simulink model "VehicleModelwithLateralController_comp"  (R2019b)
settings: Solver=FixedStepAuto  StartTime=0.0  StopTime=60  FixedStep=0.05  RelTol=1e-3
values from neighbouring files (symbols this model uses):
  Iz = car.iz    [Vehicle_Parameters_and_initial_state_comp.m]    (also in sfun_LQRwithFF_YC_2DOF.m; sfun_MPC_YC_2DOF.m; sfun_MPC_deltaU_YC_2DOF.m; sfun_MPC_deltaU_softcon_YC_2DOF.m)
  Kyf = car.kyf    [Vehicle_Parameters_and_initial_state_comp.m]    (also in sfun_LQRwithFF_YC_2DOF.m; sfun_MPC_YC_2DOF.m; sfun_MPC_deltaU_YC_2DOF.m; sfun_MPC_deltaU_softcon_YC_2DOF.m)
  Kyr = car.kyr    [Vehicle_Parameters_and_initial_state_comp.m]    (also in sfun_LQRwithFF_YC_2DOF.m; sfun_MPC_YC_2DOF.m; sfun_MPC_deltaU_YC_2DOF.m; sfun_MPC_deltaU_softcon_YC_2DOF.m)
  lf = car.lf    [Vehicle_Parameters_and_initial_state_comp.m]    (also in sfun_LQRwithFF_YC_2DOF.m; sfun_MPC_YC_2DOF.m; sfun_MPC_deltaU_YC_2DOF.m; sfun_MPC_deltaU_softcon_YC_2DOF.m)
  lr = car.lr    [Vehicle_Parameters_and_initial_state_comp.m]    (also in sfun_LQRwithFF_YC_2DOF.m; sfun_MPC_YC_2DOF.m; sfun_MPC_deltaU_YC_2DOF.m; sfun_MPC_deltaU_softcon_YC_2DOF.m)
  m = car.m    [Vehicle_Parameters_and_initial_state_comp.m]    (also in sfun_LQRwithFF_YC_2DOF.m; sfun_MPC_YC_2DOF.m; sfun_MPC_deltaU_YC_2DOF.m = 1; sfun_MPC_deltaU_softcon_YC_2DOF.m)
  Ta = a11+a22    [sfun_MPC_deltaU_softcon_YC_2DOF.m]
  Vx = 72/3.6    (= 20)    [Vehicle_Parameters_and_initial_state_comp.m]    (also in sfun_LQRwithFF_YC_2DOF.m = VehIniSt.xd; sfun_MPC_YC_2DOF.m = VehIniSt.xd; sfun_MPC_deltaU_YC_2DOF.m = VehIniSt.xd; sfun_MPC_deltaU_softcon_YC_2DOF.m = VehIniSt.xd)
  X_up = 140    [Vehicle_Parameters_and_initial_state_comp.m]
undefined symbols (not defined in the file or in its folder): car, Tra, VehIniSt
libraries: simulink x2
settings Model: Creator=pc  LastModifiedBy=YC

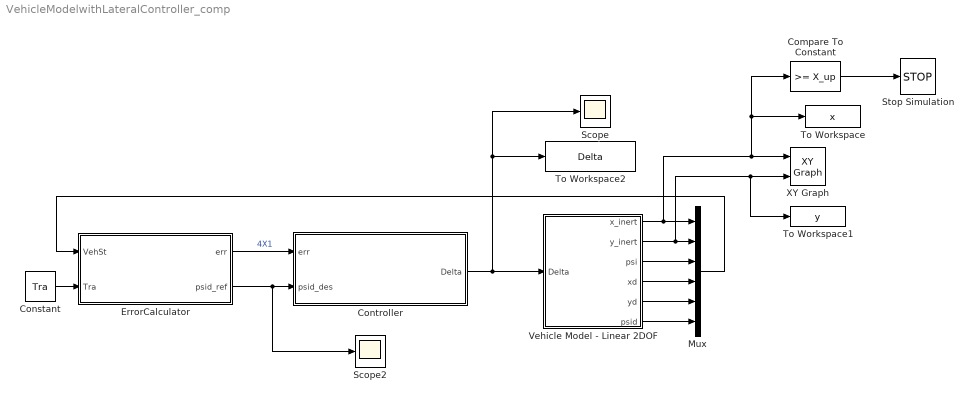
== system VehicleModelwithLateralController_comp ==
  Compare To Constant : simulink/Logic and Bit Operations/Compare To Constant  relop=>=  const=X_up  OutDataTypeStr=boolean
  Constant : Constant  Value=Tra
  Controller : Subsystem  Variant=on
  ErrorCalculator : Subsystem  Variant=on
  Mux : Mux  Inputs=6
  Scope : Scope
  Scope2 : Scope
  Stop Simulation : Stop
  To Workspace : ToWorkspace  VariableName=x  SampleTime=-1
  To Workspace1 : ToWorkspace  VariableName=y  SampleTime=-1
  To Workspace2 : ToWorkspace  VariableName=Delta  SampleTime=-1
  Vehicle Model - Linear 2DOF : Subsystem  mask{Ar=[-(2*Kyf+2*Kyr)/m/Vx,-Vx-(2*Kyf*lf-2*Kyr*lr)/m/Vx;-(2*Kyf*lf-2*Kyr*lr)/Iz/Vx,-(2*Kyf*lf.^2+2*Kyr*lr.^2)/Iz/Vx], Br=[2*Kyf/m;2*Kyf*lf/Iz], Cr=[1,0;0,1], Dr=[0;0]}
  XY Graph : simulink/Sinks/XY Graph  xmin=0  xmax=150  ymin=-1  ymax=4  st=-1
  wires:
  Compare To Constant/1 -> Stop Simulation/1
  Constant/1 -> ErrorCalculator/2(Tra)
  ErrorCalculator/1(err) -> Controller/1(err)  "4X1"
  ErrorCalculator/2(psid_ref) -> Scope2/1, Controller/2(psid_des)
  Controller/1(Delta) -> Vehicle Model - Linear 2DOF/1(Delta), Scope/1, To Workspace2/1
  Vehicle Model - Linear 2DOF/1(x_inert) -> Compare To Constant/1, To Workspace/1, XY Graph/1, Mux/1
  Vehicle Model - Linear 2DOF/2(y_inert) -> To Workspace1/1, XY Graph/2, Mux/2
  Vehicle Model - Linear 2DOF/3(psi) -> Mux/3
  Vehicle Model - Linear 2DOF/4(xd) -> Mux/4
  Vehicle Model - Linear 2DOF/5(yd) -> Mux/5
  Vehicle Model - Linear 2DOF/6(psid) -> Mux/6
  Mux/1 -> ErrorCalculator/1(VehSt)

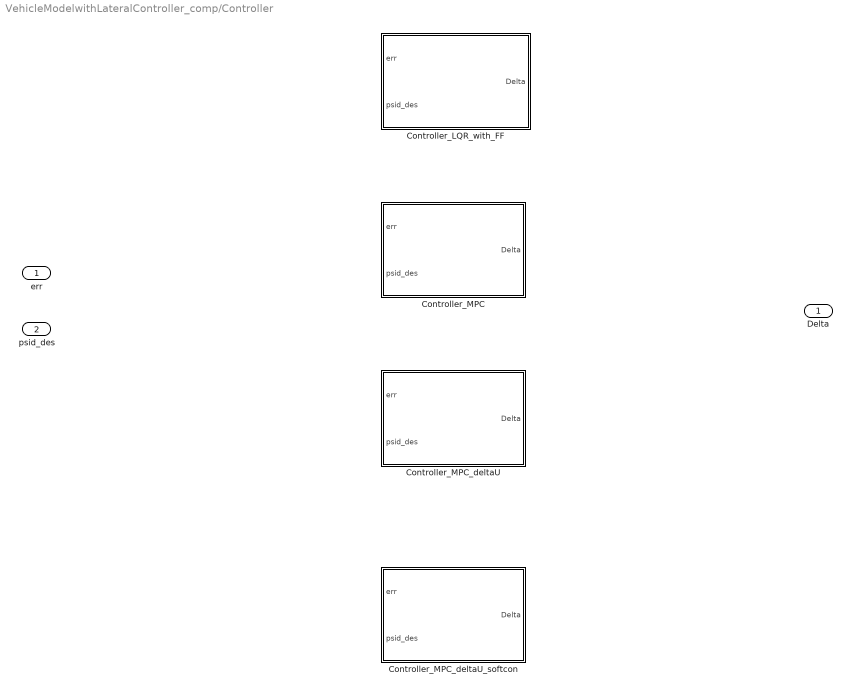
== system VehicleModelwithLateralController_comp/Controller ==
  err : Inport
  psid_des : Inport  Port=2
  Controller_LQR_with_FF : Subsystem  VariantControl=Controller_mode==1
  Controller_MPC : Subsystem  VariantControl=Controller_mode==2
  Controller_MPC_deltaU : Subsystem  VariantControl=Controller_mode==3
  Controller_MPC_deltaU_softcon : Subsystem  VariantControl=Controller_mode==4
  Delta : Outport

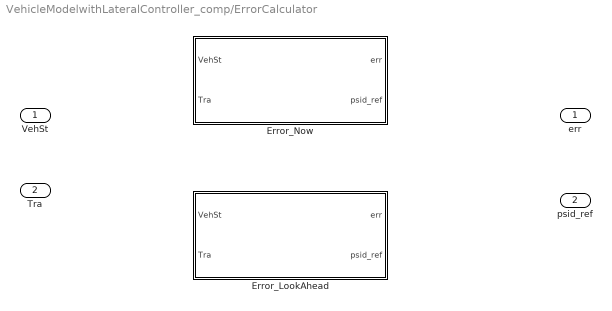
== system VehicleModelwithLateralController_comp/ErrorCalculator ==
  VehSt : Inport
  Tra : Inport  Port=2
  Error_LookAhead : Subsystem  VariantControl=Error_Mode==1
  Error_Now : Subsystem  VariantControl=Error_Mode==0
  err : Outport
  psid_ref : Outport  Port=2

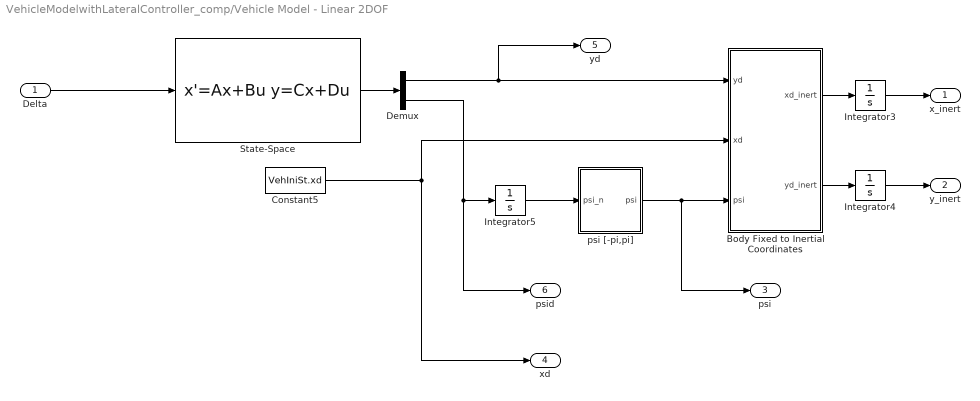
== system VehicleModelwithLateralController_comp/Vehicle Model - Linear 2DOF ==
  Delta : Inport
  Body Fixed to Inertial Coordinates : Subsystem
  Constant5 : Constant  Value=VehIniSt.xd
  Demux : Demux  Outputs=2
  Integrator3 : Integrator  InitialCondition=VehIniSt.x0
  Integrator4 : Integrator  InitialCondition=VehIniSt.y0
  Integrator5 : Integrator  InitialCondition=VehIniSt.psi0
  State-Space : StateSpace  A=Ar  B=Br  C=Cr  D=Dr  InitialCondition=0
  psi [-pi,pi] : MATLAB Function  TreatAsAtomicUnit=on
  x_inert : Outport
  y_inert : Outport  Port=2
  psi : Outport  Port=3
  xd : Outport  Port=4
  yd : Outport  Port=5
  psid : Outport  Port=6
  wires:
  Demux/2 -> Integrator5/1, psid/1
  State-Space/1 -> Demux/1
  Demux/1 -> yd/1, Body Fixed to Inertial Coordinates/1(yd)
  Delta/1 -> State-Space/1
  Body Fixed to Inertial Coordinates/2(yd_inert) -> Integrator4/1
  Integrator3/1 -> x_inert/1
  Body Fixed to Inertial Coordinates/1(xd_inert) -> Integrator3/1
  Integrator4/1 -> y_inert/1
  Constant5/1 -> xd/1, Body Fixed to Inertial Coordinates/2(xd)
  Integrator5/1 -> psi [-pi,pi]/1(psi_n)
  psi [-pi,pi]/1(psi) -> psi/1, Body Fixed to Inertial Coordinates/3(psi)

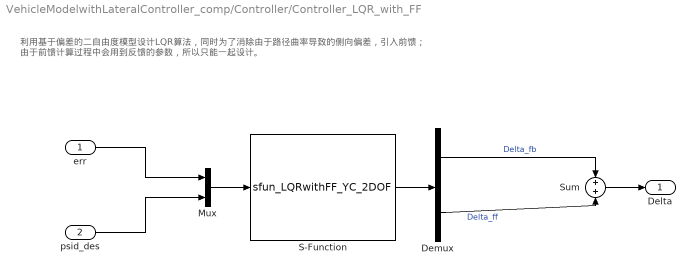
== system VehicleModelwithLateralController_comp/Controller/Controller_LQR_with_FF ==
  note: 利用基于偏差的二自由度模型设计LQR算法，同时为了消除由于路径曲率导致的侧向偏差，引入前馈；
      | 由于前馈计算过程中会用到反馈的参数，所以只能一起设计。
  err : Inport
  psid_des : Inport  Port=2
  Demux : Demux  Outputs=2
  Mux : Mux  Inputs=2
  S-Function : S-Function  FunctionName=sfun_LQRwithFF_YC_2DOF  Parameters=car,VehIniSt  SFunctionDeploymentMode=off  EnableBusSupport=off
  Sum : Sum  Inputs=+|+
  Delta : Outport
  wires:
  Mux/1 -> S-Function/1
  err/1 -> Mux/1
  psid_des/1 -> Mux/2
  Demux/2 -> Sum/2  "Delta_ff"
  Demux/1 -> Sum/1  "Delta_fb"
  Sum/1 -> Delta/1
  S-Function/1 -> Demux/1

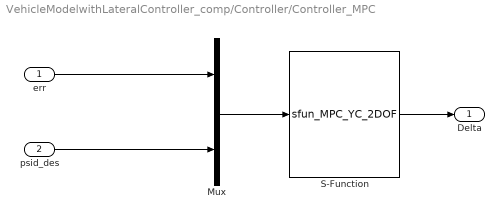
== system VehicleModelwithLateralController_comp/Controller/Controller_MPC ==
  err : Inport
  psid_des : Inport  Port=2
  Mux : Mux  Inputs=2
  S-Function : S-Function  FunctionName=sfun_MPC_YC_2DOF  Parameters=car,VehIniSt  SFunctionDeploymentMode=off  EnableBusSupport=off
  Delta : Outport
  wires:
  psid_des/1 -> Mux/2
  S-Function/1 -> Delta/1
  err/1 -> Mux/1
  Mux/1 -> S-Function/1

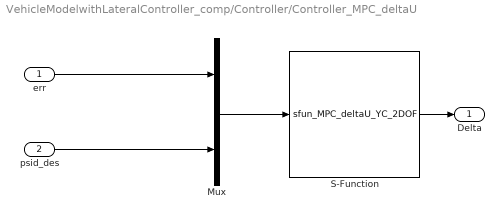
== system VehicleModelwithLateralController_comp/Controller/Controller_MPC_deltaU ==
  err : Inport
  psid_des : Inport  Port=2
  Mux : Mux  Inputs=2
  S-Function : S-Function  FunctionName=sfun_MPC_deltaU_YC_2DOF  Parameters=car,VehIniSt  SFunctionDeploymentMode=off  EnableBusSupport=off
  Delta : Outport
  wires:
  psid_des/1 -> Mux/2
  S-Function/1 -> Delta/1
  err/1 -> Mux/1
  Mux/1 -> S-Function/1

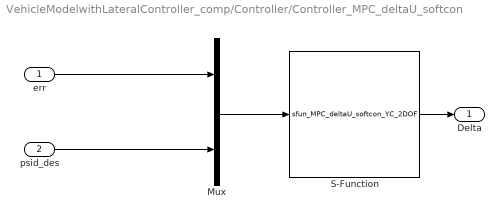
== system VehicleModelwithLateralController_comp/Controller/Controller_MPC_deltaU_softcon ==
  err : Inport
  psid_des : Inport  Port=2
  Mux : Mux  Inputs=2
  S-Function : S-Function  FunctionName=sfun_MPC_deltaU_softcon_YC_2DOF  Parameters=car,VehIniSt  SFunctionDeploymentMode=off  EnableBusSupport=off
  Delta : Outport
  wires:
  psid_des/1 -> Mux/2
  S-Function/1 -> Delta/1
  err/1 -> Mux/1
  Mux/1 -> S-Function/1

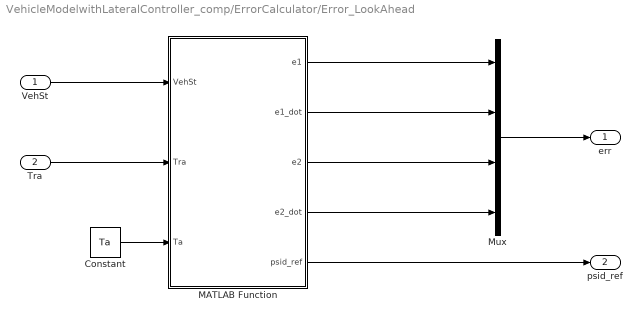
== system VehicleModelwithLateralController_comp/ErrorCalculator/Error_LookAhead ==
  VehSt : Inport
  Tra : Inport  Port=2
  Constant : Constant  Value=Ta
  MATLAB Function : MATLAB Function  TreatAsAtomicUnit=on
  Mux : Mux
  err : Outport
  psid_ref : Outport  Port=2
  wires:
  MATLAB Function/2(e1_dot) -> Mux/2
  MATLAB Function/3(e2) -> Mux/3
  Mux/1 -> err/1
  MATLAB Function/1(e1) -> Mux/1
  Tra/1 -> MATLAB Function/2(Tra)
  MATLAB Function/4(e2_dot) -> Mux/4
  MATLAB Function/5(psid_ref) -> psid_ref/1
  VehSt/1 -> MATLAB Function/1(VehSt)
  Constant/1 -> MATLAB Function/3(Ta)

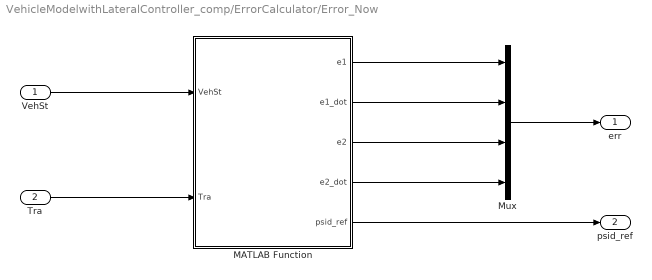
== system VehicleModelwithLateralController_comp/ErrorCalculator/Error_Now ==
  VehSt : Inport
  Tra : Inport  Port=2
  MATLAB Function : MATLAB Function  TreatAsAtomicUnit=on
  Mux : Mux
  err : Outport
  psid_ref : Outport  Port=2
  wires:
  MATLAB Function/2(e1_dot) -> Mux/2
  MATLAB Function/3(e2) -> Mux/3
  Mux/1 -> err/1
  MATLAB Function/1(e1) -> Mux/1
  Tra/1 -> MATLAB Function/2(Tra)
  MATLAB Function/4(e2_dot) -> Mux/4
  MATLAB Function/5(psid_ref) -> psid_ref/1
  VehSt/1 -> MATLAB Function/1(VehSt)

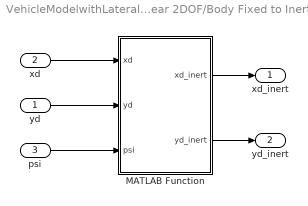
== system VehicleModelwithLateralController_comp/Vehicle Model - Linear 2DOF/Body Fixed to Inertial Coordinates ==
  yd : Inport
  xd : Inport  Port=2
  psi : Inport  Port=3
  MATLAB Function : MATLAB Function  TreatAsAtomicUnit=on
  xd_inert : Outport
  yd_inert : Outport  Port=2
  wires:
  MATLAB Function/1(xd_inert) -> xd_inert/1
  MATLAB Function/2(yd_inert) -> yd_inert/1
  xd/1 -> MATLAB Function/1(xd)
  yd/1 -> MATLAB Function/2(yd)
  psi/1 -> MATLAB Function/3(psi)

== matlab function VehicleModelwithLateralController_comp/Vehicle Model - Linear 2DOF/Body Fixed to Inertial Coordinates/MATLAB Function ==
  data: xd input; yd input; psi input; xd_inert output; yd_inert output
function [xd_inert,yd_inert] = fcn(xd,yd,psi)

xd_inert=xd.*cos(psi)-yd.*sin(psi);
yd_inert=xd.*sin(psi)+yd.*cos(psi);
end

== matlab function VehicleModelwithLateralController_comp/ErrorCalculator/Error_Now/MATLAB Function ==
  data: VehSt input; Tra input; e1 output; e1_dot output; e2 output; e2_dot output; psid_ref output
function [e1,e1_dot,e2,e2_dot,psid_ref] = fcn(VehSt,Tra)
% % x_ref,y_ref,psi_ref,kappa_ref,n是调试用的，检验这个函数的正确性。已删除

% 车辆实时状态
x_inert=VehSt(1);
y_inert=VehSt(2);
psi=VehSt(3);
Vx=VehSt(4);
yd=VehSt(5);
psid=VehSt(6);
% 规划轨迹
X=Tra(:,1);
Y=Tra(:,2);
PSI=Tra(:,3);
KAPPA=Tra(:,4);

% 寻找距离最近点nearest_point
dX=x_inert-X;
dY=y_inert-Y;
deltaS=sqrt(dX.^2+dY.^2);
[~,n]=min(deltaS);% 索引为n的点即为距离最近点

% % 偏差计算,直接根据距离最近点算偏差，目前来说效果不太好，放弃。
% x_ref=X(n);y_ref=Y(n);
% e1=(y_inert-y_ref).*cos(PSI(n))-(x_inert-x_ref).*sin(PSI(n));
% e2=psi-PSI(n);
% e1_dot=Vx.*sin(e2);
% e2_dot=psid-Vx.*KAPPA(n);
% psid_ref=Vx.*KAPPA(n);
% %*************************测试用
% psi_ref=PSI(n);
% kappa_ref=KAPPA(n);
% %******************************


% 偏差计算，在最近点和下一个点的基础上找投影点
if n==length(X) %防止到最后一个点还找一下个点，产生超出
    x_ref = X(n);
    y_ref = Y(n);
    psi_ref =PSI(n);
    kappa_ref =KAPPA(n);
else 
    tol=0.001;
    if abs(X(n+1)-X(n))<tol %直线PnPn+1斜率很大
        x_proj = X(n);
        y_proj = y_inert;
    elseif abs(Y(n+1)-Y(n))<tol %直线PnPn+1斜率为零
        x_proj = x_inert;
        y_proj = Y(n);
    else
        k1=(Y(n+1)-Y(n))/(X(n+1)-X(n));%直线PnPn+1斜率
        k2=-1/k1;
        x_proj = (y_inert-Y(n)+k1*X(n)-k2*x_inert)/(k1-k2);% 根据两条直线的斜率和点方程求投影点
        y_proj = y_inert+k2*(x_proj-x_inert);
    end
    % 将投影点作为最终参考点
    x_ref = x_proj;
    y_ref = y_proj;
    
    dist = sqrt((X(n+1)-X(n))^2+(Y(n+1)-Y(n))^2);
    dist_p = sqrt((X(n+1)-x_proj)^2+(Y(n+1)-y_proj)^2);
    ratio = dist_p/dist;
    psi_ref = ratio*PSI(n)+(1-ratio)*PSI(n+1);
    kappa_ref = ratio*KAPPA(n)+(1-ratio)*KAPPA(n+1);
end
% 偏差计算,以参考轨迹坐标系计算偏差,当前点与参考点的差值（当前点在前，与基于偏差的动力学模型保持一致）
e1=(y_inert-y_ref).*cos(psi_ref)-(x_inert-x_ref).*sin(psi_ref);
% e1=(y_inert-y_ref).*cos(psi)-(x_inert-x_ref).*sin(psi);
e2=psi-psi_ref;
if e2<=-pi % 因为psi是(-pi,pi]，是有界的,防止越界时在-pi,pi之间反复越界跳
    e2=2*pi+e2;
elseif e2>pi
    e2=e2-2*pi;
end
e1_dot=Vx.*sin(e2);
% e1_dot=yd+Vx*e2;
e2_dot=psid-Vx.*kappa_ref;
psid_ref=Vx.*kappa_ref;
    
end

== matlab function VehicleModelwithLateralController_comp/Vehicle Model - Linear 2DOF/psi [-pi,pi] ==
  data: psi_n input; psi output
function psi = fcn(psi_n)

psi=mod(psi_n,2*pi);
if psi>pi
    psi = psi-2*pi;
end

end

== matlab function VehicleModelwithLateralController_comp/ErrorCalculator/Error_LookAhead/MATLAB Function ==
  data: VehSt input; Tra input; e1 output; e1_dot output; e2 output; e2_dot output; psid_ref output; Ta input
function [e1,e1_dot,e2,e2_dot,psid_ref] = fcn(VehSt,Tra,Ta)
% 车辆实时状态
x_inert=VehSt(1);
y_inert=VehSt(2);
psi=VehSt(3);
Vx=VehSt(4);
yd=VehSt(5);
psid=VehSt(6);
% 规划轨迹
X=Tra(:,1);
Y=Tra(:,2);
PSI=Tra(:,3);
KAPPA=Tra(:,4);

% 寻找距离最近点nearest_point
dX=x_inert-X;
dY=y_inert-Y;
deltaS=sqrt(dX.^2+dY.^2);
[~,n]=min(deltaS);% 索引为n的点即为距离最近点

% 偏差计算，在最近点和下一个点的基础上找投影点（比最近点更近的点）
tol=0.001;
if abs(X(n+1)-X(n))<tol %直线PnPn+1斜率很大
    x_proj = X(n);
    y_proj = y_inert;
elseif abs(Y(n+1)-Y(n))<tol %直线PnPn+1斜率为零
    x_proj = x_inert;
    y_proj = Y(n);
else
    k1=(Y(n+1)-Y(n))/(X(n+1)-X(n));%直线PnPn+1斜率
    k2=-1/k1;
    x_proj = (y_inert-Y(n)+k1*X(n)-k2*x_inert)/(k1-k2);% 根据两条直线的斜率和点方程求投影点
    y_proj = y_inert+k2*(x_proj-x_inert);
end

dist_p = sqrt((X(n+1)-x_proj)^2+(Y(n+1)-y_proj)^2);
% 在投影点以及参考轨迹的基础上做预瞄，找预瞄参考点
for m=n+1:length(X)-1 % 有超出终点的风险 
    if dist_p-Vx*Ta<0
        dist_p = dist_p+sqrt((X(m+1)-X(m))^2+(Y(m+1)-Y(m))^2);
    else
        break;
    end
end
dist_q = dist_p-Vx*Ta;% 相对m点往回多远距离
dist_r = sqrt((X(m-1)-X(m))^2+(Y(m-1)-Y(m))^2);% m和m-1点之间的距离
ratio1 = dist_q/dist_r;

x_ref = X(m)-ratio1*(X(m)-X(m-1));% 预瞄参考点
y_ref = Y(m)-ratio1*(Y(m)-Y(m-1));
psi_ref = ratio1*PSI(m-1)+(1-ratio1)*PSI(m);
kappa_ref = ratio1*KAPPA(m-1)+(1-ratio1)*KAPPA(m);

% 偏差计算,以参考轨迹坐标系计算偏差,当前点Ta时间后与预瞄参考点的差值（当前点在前，与基于偏差的动力学模型保持一致）
e1=(y_inert-y_ref).*cos(psi_ref)-(x_inert-x_ref).*sin(psi_ref);
% e1=(y_inert-y_ref).*cos(psi)-(x_inert-x_ref).*sin(psi);
e2=psi-psi_ref;
if e2<=-pi % 因为psi是(-pi,pi]，是有界的,防止越界时在-pi,pi之间反复横跳
    e2=2*pi+e2;
elseif e2>pi
    e2=e2-2*pi;
end
e1_dot=Vx.*sin(e2);
% e1_dot=yd+Vx*e2;
e2_dot=psid-Vx.*kappa_ref;
psid_ref=Vx.*kappa_ref;
%预瞄
% e1=e1+Vx*Ta*sin(psid*Ta/2+yd/Vx);% 考虑到车辆的平动和旋转，但是近似的
e1=e1+Vx*Ta*sin(yd/Vx); % 仅考虑车辆的平动
e2=e2+psid*Ta; 
end
